simulink model "pid_test_model"  (Simulink 8.3)
settings: Solver=ode45  StartTime=0.0  StopTime=50  RelTol=1e-3
libraries: simulink x2
settings Model: Creator=Yura  LastModifiedBy=Yura
settings DataIOCC: SignalLoggingSaveFormat=Dataset
settings DebuggingCC: UnderspecifiedInitializationDetection=Simplified  StateNameClashWarn=none
settings GRTTargetCC: CombineOutputUpdateFcns=on  GRTInterface=off

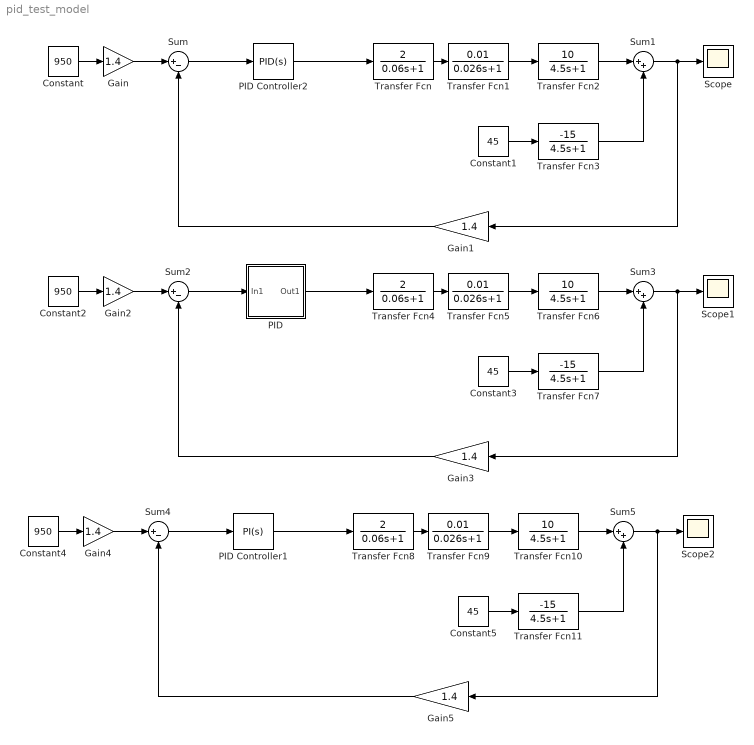
== system pid_test_model ==
  Constant : Constant  Value=950
  Constant1 : Constant  Value=45
  Constant2 : Constant  Value=950
  Constant3 : Constant  Value=45
  Constant4 : Constant  Value=950
  Constant5 : Constant  Value=45
  Gain{,1..5} (6 alike) : Gain  Gain=1.4
  PID : Subsystem
  PID Controller1 : simulink/Continuous/PID Controller  Controller=PI  TimeDomain=Continuous-time  SampleTime=1  IntegratorMethod=Forward Euler  FilterMethod=Forward Euler  Form=Parallel  P=2.15472953690211  I=1.43865449702428  D=-9.46783887166763  N=0.392320719070336  InitialConditionSource=internal  InitialConditionForIntegrator=0  InitialConditionForFilter=0  ExternalReset=none  LimitOutput=off  UpperSaturationLimit=inf  LowerSaturationLimit=-inf  LinearizeAsGain=on  AntiWindupMode=none  Kb=1  TrackingMode=off  Kt=1  PParamMin=[]  PParamMax=[]  IParamMin=[]  IParamMax=[]  DParamMin=[]  DParamMax=[]  NParamMin=[]  NParamMax=[]  KbParamMin=[]  KbParamMax=[]  KtParamMin=[]  KtParamMax=[]  POutMin=[]  POutMax=[]  IOutMin=[]  IOutMax=[]  DOutMin=[]  DOutMax=[]  NOutMin=[]  NOutMax=[]  KbOutMin=[]  KbOutMax=[]  KtOutMin=[]  KtOutMax=[]  IntegratorOutMin=[]  IntegratorOutMax=[]  FilterOutMin=[]  FilterOutMax=[]  SumOutMin=[]  SumOutMax=[]  SumI1OutMin=[]  SumI1OutMax=[]  SumI2OutMin=[]  SumI2OutMax=[]  SumI3OutMin=[]  SumI3OutMax=[]  SumDOutMin=[]  SumDOutMax=[]  SaturationOutMin=[]  SaturationOutMax=[]  IntegratorContinuousStateAttributes=''  IntegratorStateMustResolveToSignalObject=off  IntegratorRTWStateStorageClass=Auto  FilterContinuousStateAttributes=''  FilterStateMustResolveToSignalObject=off  FilterRTWStateStorageClass=Auto
  PID Controller2 : simulink/Continuous/PID Controller  Controller=PID  TimeDomain=Continuous-time  SampleTime=1  IntegratorMethod=Forward Euler  FilterMethod=Forward Euler  Form=Parallel  P=5.74176336474208  I=1.67239560209647  D=-9.46783887166763  N=0.392320719070336  InitialConditionSource=internal  InitialConditionForIntegrator=0  InitialConditionForFilter=0  ExternalReset=none  LimitOutput=off  UpperSaturationLimit=inf  LowerSaturationLimit=-inf  LinearizeAsGain=on  AntiWindupMode=none  Kb=1  TrackingMode=off  Kt=1  PParamMin=[]  PParamMax=[]  IParamMin=[]  IParamMax=[]  DParamMin=[]  DParamMax=[]  NParamMin=[]  NParamMax=[]  KbParamMin=[]  KbParamMax=[]  KtParamMin=[]  KtParamMax=[]  POutMin=[]  POutMax=[]  IOutMin=[]  IOutMax=[]  DOutMin=[]  DOutMax=[]  NOutMin=[]  NOutMax=[]  KbOutMin=[]  KbOutMax=[]  KtOutMin=[]  KtOutMax=[]  IntegratorOutMin=[]  IntegratorOutMax=[]  FilterOutMin=[]  FilterOutMax=[]  SumOutMin=[]  SumOutMax=[]  SumI1OutMin=[]  SumI1OutMax=[]  SumI2OutMin=[]  SumI2OutMax=[]  SumI3OutMin=[]  SumI3OutMax=[]  SumDOutMin=[]  SumDOutMax=[]  SaturationOutMin=[]  SaturationOutMax=[]  IntegratorContinuousStateAttributes=''  IntegratorStateMustResolveToSignalObject=off  IntegratorRTWStateStorageClass=Auto  FilterContinuousStateAttributes=''  FilterStateMustResolveToSignalObject=off  FilterRTWStateStorageClass=Auto
  Scope : Scope
      settings: TickLabels=on  ShowLegends=on  SampleInput=on
  Scope1 : Scope
      settings: TickLabels=on  ShowLegends=on  SampleInput=on
  Scope2 : Scope
      settings: TickLabels=on  ShowLegends=on  SaveName=ScopeData2  SampleInput=on
  Sum : Sum  Inputs=|+-
  Sum1 : Sum  Inputs=|++
  Sum2 : Sum  Inputs=|+-
  Sum3 : Sum  Inputs=|++
  Sum4 : Sum  Inputs=|+-
  Sum5 : Sum  Inputs=|++
  Transfer Fcn : TransferFcn  Numerator=[2]  Denominator=[0.06 1]
  Transfer Fcn1 : TransferFcn  Numerator=[0.01]  Denominator=[0.026 1]
  Transfer Fcn10 : TransferFcn  Numerator=[10]  Denominator=[4.5 1]
  Transfer Fcn11 : TransferFcn  Numerator=[-15]  Denominator=[4.5 1]
  Transfer Fcn2 : TransferFcn  Numerator=[10]  Denominator=[4.5 1]
  Transfer Fcn3 : TransferFcn  Numerator=[-15]  Denominator=[4.5 1]
  Transfer Fcn4 : TransferFcn  Numerator=[2]  Denominator=[0.06 1]
  Transfer Fcn5 : TransferFcn  Numerator=[0.01]  Denominator=[0.026 1]
  Transfer Fcn6 : TransferFcn  Numerator=[10]  Denominator=[4.5 1]
  Transfer Fcn7 : TransferFcn  Numerator=[-15]  Denominator=[4.5 1]
  Transfer Fcn8 : TransferFcn  Numerator=[2]  Denominator=[0.06 1]
  Transfer Fcn9 : TransferFcn  Numerator=[0.01]  Denominator=[0.026 1]
  wires:
  Constant/1 -> Gain/1
  Gain/1 -> Sum/1
  Transfer Fcn/1 -> Transfer Fcn1/1
  Transfer Fcn1/1 -> Transfer Fcn2/1
  Transfer Fcn2/1 -> Sum1/1
  Sum1/1 -> Gain1/1, Scope/1
  Transfer Fcn3/1 -> Sum1/2
  Constant1/1 -> Transfer Fcn3/1
  Gain1/1 -> Sum/2
  Sum/1 -> PID Controller2/1
  PID Controller2/1 -> Transfer Fcn/1
  Constant2/1 -> Gain2/1
  Gain2/1 -> Sum2/1
  Transfer Fcn4/1 -> Transfer Fcn5/1
  Transfer Fcn5/1 -> Transfer Fcn6/1
  Transfer Fcn6/1 -> Sum3/1
  Sum3/1 -> Scope1/1, Gain3/1
  Transfer Fcn7/1 -> Sum3/2
  Constant3/1 -> Transfer Fcn7/1
  Gain3/1 -> Sum2/2
  Sum2/1 -> PID/1(In1)
  PID/1(Out1) -> Transfer Fcn4/1
  Constant4/1 -> Gain4/1
  Gain4/1 -> Sum4/1
  Transfer Fcn8/1 -> Transfer Fcn9/1
  Transfer Fcn9/1 -> Transfer Fcn10/1
  Transfer Fcn10/1 -> Sum5/1
  Sum5/1 -> Scope2/1, Gain5/1
  Transfer Fcn11/1 -> Sum5/2
  Constant5/1 -> Transfer Fcn11/1
  Gain5/1 -> Sum4/2
  Sum4/1 -> PID Controller1/1
  PID Controller1/1 -> Transfer Fcn8/1

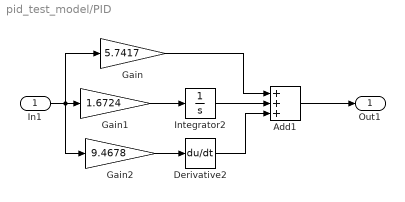
== system pid_test_model/PID ==
  In1 : Inport
  Add1 : Sum  Inputs=+++
  Derivative2 : Derivative
  Gain : Gain  Gain=5.7417
  Gain1 : Gain  Gain=1.6724
  Gain2 : Gain  Gain=9.4678
  Integrator2 : Integrator
  Out1 : Outport
  wires:
  Gain1/1 -> Integrator2/1
  Add1/1 -> Out1/1
  Gain/1 -> Add1/1
  In1/1 -> Gain1/1, Gain/1, Gain2/1
  Gain2/1 -> Derivative2/1
  Derivative2/1 -> Add1/3
  Integrator2/1 -> Add1/2
